simulink model "Velocity"  (R2019a)
settings: Solver=FixedStepDiscrete  StartTime=0.0  StopTime=100  FixedStep=1  RelTol=1e-3
values from neighbouring files (symbols this model uses):
  Pressure = 1800.0 1650.0 1500.0 1350.0 1200.0 1050.0 900.0 750.0 600.0 450.0 300.0    [fomulaM.sldd]
settings Model: DataDictionary=fomulaM.sldd  Creator=Admin  LastModifiedBy=Admin

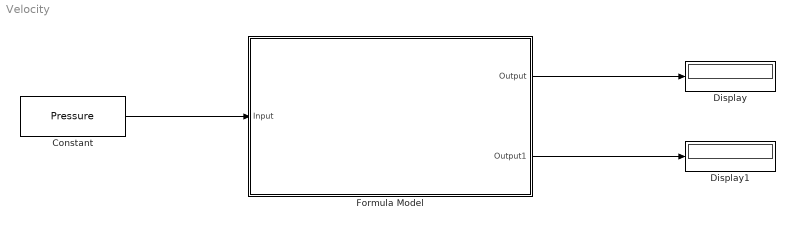
== system Velocity ==
  Constant : Constant  Value=Pressure
  Display : Display
  Display1 : Display
  "Formula Model " : Subsystem
  wires:
  "Formula Model "/1(Output) -> Display/1
  "Formula Model "/2(Output1) -> Display1/1
  Constant/1 -> "Formula Model "/1(Input)

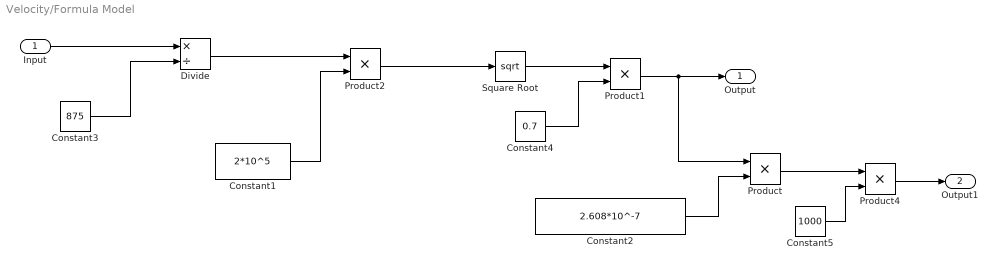
== system Velocity/Formula Model  ==
  Input : Inport
  Constant1 : Constant  Value=2*10^5
  Constant2 : Constant  Value=2.608*10^-7
  Constant3 : Constant  Value=875
  Constant4 : Constant  Value=0.7
  Constant5 : Constant  Value=1000
  Divide : Product  Inputs=*/
  Product{,1..2,4} (4 alike) : Product
  Square Root : Sqrt  SaturateOnIntegerOverflow=on
  Output : Outport
  Output1 : Outport  Port=2
  wires:
  Square Root/1 -> Product1/1
  Constant4/1 -> Product1/2
  Constant3/1 -> Divide/2
  Constant1/1 -> Product2/2
  Divide/1 -> Product2/1
  Product2/1 -> Square Root/1
  Product1/1 -> Product/1, Output/1
  Input/1 -> Divide/1
  Constant2/1 -> Product/2
  Product/1 -> Product4/1
  Product4/1 -> Output1/1
  Constant5/1 -> Product4/2
